simulink model "simModel2020"  (R2023b)
settings: Solver=ode4  StartTime=0  StopTime=360  FixedStep=0.01  RelTol=1e-3
values from neighbouring files (symbols this model uses):
  B747 =     [B747.mat]
undefined symbols (not defined in the file or in its folder): airport, APP, control, Curise, Earth, env, ft, m, navData, navParam, Newton, plotTrack, Raphson, s, TakeOff, WGS84
libraries: aerolibconvert2 x18, simulink x15, sharedtransform x4, aerolibfltsims x3, aerolibatmos2 x2, shared6dof x2, aerolibasang x2, dspsrcs4 x2, aerolibwind2 x2, aerolibanimutils x1, aerolibpropulsion2 x1, aerolibtransform2 x1
(part 5 of 6)

== system simModel2020/AutoPilot/InnerLoopAutopilot/Longitudinal Channel经度通道/AutoThrottle/AT Mode = 5,Idle/Rate Limiter Dynamic with External IC and Autoreset for Change in IC/Saturation Dynamic ==
  up : Inport
  u : Inport  Port=2
  lo : Inport  Port=3
  Data Type Duplicate : DataTypeDuplicate  DisableCoverage=on
  Data Type Propagation : S-Function  FunctionName=sfix_dtprop  Parameters=14,PropDataTypeMode,(getdatatypespecs(PropDataType,PropScaling,DblOver,0, 0, PropDataTypeMode, PropScalingMode)),IfRefDouble,IfRefSingle,IsSigned,NumBitsBase,NumBitsMult,NumBitsAdd,(sort(reshape(round(NumBitsAllowFinal), prod(size(NumBitsAllowFinal)),1))),PropScalingMode,ValuesUsedBestPrec,SlopeBase,SlopeMult,SlopeAdd,BiasBase,BiasMult,BiasAdd,DblOver  SFunctionDeploymentMode=off  EnableBusSupport=off  mask(Data Type Propagation){PropDataTypeMode=Inherit via propagation rule, PropDataType=fixdt(1, 16), IfRefDouble=double, IfRefSingle=single, IsSigned=IsSigned1, NumBitsBase=NumBits1, NumBitsMult=1, NumBitsAdd=0, NumBitsAllowFinal=1:128, PropScalingMode=Inherit via propagation rule, PropScaling=2^-10, ValuesUsedBestPrec=[5 -7], SlopeBase=Slope1, SlopeMult=1, SlopeAdd=0, BiasBase=Bias1, BiasMult=1, BiasAdd=0}
      mask prompts: PropDataTypeMode "Simulink:masks:x1PropagatedDataType_MP"; PropDataType "Simulink:masks:x11PropagatedDataTypeegFixdt116Fixdtsingle_MP"; IfRefDouble "Simulink:masks:x11IfAnyReferenceInputIsDoubleOutputIs_MP"; IfRefSingle "Simulink:masks:x12IfAnyReferenceInputIsSingleOutputIs_MP"; IsSigned "Simulink:masks:x13IsSigned_MP"; NumBitsBase "Simulink:masks:x141NumberofBitsBase_MP"; NumBitsMult "Simulink:masks:x142NumberofBitsMultiplicativeAdjustment_MP"; NumBitsAdd "Simulink:masks:x143NumberofBitsAdditiveAdjustment_MP"; NumBitsAllowFinal "Simulink:masks:x144NumberofBitsAllowableFinalValues_MP"; PropScalingMode "Simulink:masks:x2PropagatedScaling_MP"; PropScaling "Simulink:masks:x21PropagatedScalingSlopeEg29OrSlopeBiasEg1253_MP"; ValuesUsedBestPrec "Simulink:masks:x21ValuesUsedToDetermineBestPrecisionScaling_MP"; SlopeBase "Simulink:masks:x211SlopeBase_MP"; SlopeMult "Simulink:masks:x212SlopeMultiplicativeAdjustment_MP"; SlopeAdd "Simulink:masks:x213SlopeAdditiveAdjustment_MP"; BiasBase "Simulink:masks:x221BiasBase_MP"; BiasMult "Simulink:masks:x222BiasMultiplicativeAdjustment_MP"; BiasAdd "Simulink:masks:x223BiasAdditiveAdjustment_MP"
      mask help: Simulink:masks:DataTypePropagation_MD
      mask init:
      | DblOver = 0;
      mask TypeOptions PropDataTypeMode: Simulink:masks:SpecifyViaDialog | Simulink:masks:InheritViaPropagationRule
      mask Callback PropDataTypeMode: fixptdialog(gcbh)
      mask Callback PropDataType: fixptdialog(gcbh)
      mask TypeOptions IfRefDouble: Simulink:masks:double | Simulink:masks:single
      mask TypeOptions IfRefSingle: Simulink:masks:double | Simulink:masks:single
      mask TypeOptions IsSigned: Simulink:masks:IsSigned1 | Simulink:masks:IsSigned2 | Simulink:masks:IsSigned1OrIsSigned2 | Simulink:masks:TRUE | Simulink:masks:FALSE
      mask TypeOptions NumBitsBase: NumBits1 | NumBits2 | max([NumBits1 NumBits2]) | min([NumBits1 NumBits2]) | NumBits1+NumBits2
      mask TypeOptions PropScalingMode: Simulink:masks:SpecifyViaDialog | Simulink:masks:InheritViaPropagationRule | Simulink:masks:ObtainViaBestPrecision
      mask Callback PropScalingMode: fixptdialog(gcbh)
      mask TypeOptions SlopeBase: Slope1 | Slope2 | max([Slope1 Slope2]) | min([Slope1 Slope2]) | Slope1*Slope2 | Slope1/Slope2 | PosRange1 | PosRange2 | max([PosRange1 PosRange2]) | min([PosRange1 PosRange2]) | PosRange1*PosRange2 | PosRange1/PosRange2
      mask TypeOptions BiasBase: Bias1 | Bias2 | max([Bias1 Bias2]) | min([Bias1 Bias2]) | Bias1*Bias2 | Bias1/Bias2 | Bias1+Bias2 | Bias1-Bias2
      mask Display:
      | port_label('Input',1,'Ref1');
      | port_label('Input',2,'Ref2');
      | port_label('Input',3,'Prop');
  LowerRelop1 : RelationalOperator  DisableCoverage=on  Operator=>  OutDataTypeStr=boolean  InputSameDT=off
  Switch : Switch  Criteria=u2 ~= 0  OutDataTypeStr=Inherit: Inherit via back propagation  ZeroCross=off  SaturateOnIntegerOverflow=off  InputSameDT=off
  Switch2 : Switch  Criteria=u2 ~= 0  OutMin=OutMin  OutMax=OutMax  OutDataTypeStr=Inherit: Inherit via back propagation  ZeroCross=off  SaturateOnIntegerOverflow=off  InputSameDT=off
  UpperRelop : RelationalOperator  DisableCoverage=on  Operator=<  OutDataTypeStr=boolean  InputSameDT=off
  y : Outport  OutMin=OutMin  OutMax=OutMax
  wires:
  up/1 -> Switch2/1, LowerRelop1/2
  u/1 -> Data Type Propagation/2, Data Type Propagation/1, LowerRelop1/1, Switch/3, UpperRelop/1
  lo/1 -> Switch/1, UpperRelop/2
  Switch/1 -> Data Type Duplicate/2, Switch2/3, Data Type Propagation/3
  Switch2/1 -> Data Type Duplicate/1, y/1
  LowerRelop1/1 -> Switch2/2
  UpperRelop/1 -> Switch/2

== system simModel2020/AutoPilot/InnerLoopAutopilot/Longitudinal Channel经度通道/AutoThrottle/AT Mode = 5,Idle/Rate Limiter Dynamic with External IC and Autoreset for Change in IC/Subsystem ==
  WP Fly : Inport
  Compare To Constant : Subsystem  mask(Compare To Constant){relop=>=, const=0.5, OutDataTypeStr=boolean, ZeroCross=on}
      mask prompts: relop "Simulink:masks:Operator_MP"; const "Simulink:masks:ConstantValue_MP"; OutDataTypeStr "Simulink:masks:OutputDataType_MP"; ZeroCross "Simulink:masks:EnableZerocrossingDetection_MP"
      mask help: Simulink:masks:CompareToConstant_MD
      mask init: same as simModel2020/AutoPilot/InnerLoopAutopilot/Longitudinal Channel经度通道/AutoThrottle/AT Mode = 0,Recycle/Rate Limiter Dynamic with External IC and Autoreset for Change in IC/Subsystem/Compare To Constant
      mask TypeOptions relop: == | ~= | < | <= | >= | >
      mask TypeOptions OutDataTypeStr: Simulink:masks:uint8 | Simulink:masks:boolean
      mask Callback ZeroCross: sl('zeroCrossEnable', gcbh);
      mask Display: disp(str)
  Compare To Constant1 : Subsystem  mask(Compare To Constant){relop=<, const=0.5, OutDataTypeStr=boolean, ZeroCross=on}
      mask prompts: relop "Simulink:masks:Operator_MP"; const "Simulink:masks:ConstantValue_MP"; OutDataTypeStr "Simulink:masks:OutputDataType_MP"; ZeroCross "Simulink:masks:EnableZerocrossingDetection_MP"
      mask help: Simulink:masks:CompareToConstant_MD
      mask init: same as simModel2020/AutoPilot/InnerLoopAutopilot/Longitudinal Channel经度通道/AutoThrottle/AT Mode = 0,Recycle/Rate Limiter Dynamic with External IC and Autoreset for Change in IC/Subsystem/Compare To Constant
      mask TypeOptions relop: == | ~= | < | <= | >= | >
      mask TypeOptions OutDataTypeStr: Simulink:masks:uint8 | Simulink:masks:boolean
      mask Callback ZeroCross: sl('zeroCrossEnable', gcbh);
      mask Display: disp(str)
  Logical Operator : Logic  AllPortsSameDT=off  OutDataTypeStr=boolean
  Unit Delay : UnitDelay  SampleTime=-1  HasFrameUpgradeWarning=on
  Just Enab : Outport
  wires:
  WP Fly/1 -> Unit Delay/1, Compare To Constant/1(u)
  Compare To Constant/1(y) -> Logical Operator/1
  Compare To Constant1/1(y) -> Logical Operator/2
  Unit Delay/1 -> Compare To Constant1/1(u)
  Logical Operator/1 -> Just Enab/1

== system simModel2020/AutoPilot/InnerLoopAutopilot/Longitudinal Channel经度通道/AutoThrottle/AT Mode = 5,Idle/Rate Limiter Dynamic with External IC and Autoreset for Change in IC/Unit Delay Resettable External IC ==
  note: Reset
  note: Initial Value
  u : Inport
  R : Inport  Port=2
  IC : Inport  Port=3
  FixPt Constant : Constant  DisableCoverage=on  Value=0  OutDataTypeStr=fixdt(0,8,0)
  FixPt Data Type Duplicate1 : DataTypeDuplicate  DisableCoverage=on  NumInputPorts=4
  FixPt Logical Operator : Logic  DisableCoverage=on  Operator=OR  AllPortsSameDT=off  OutDataTypeStr=fixdt(0, 8)
  FixPt Unit Delay1 : UnitDelay  DisableCoverage=on  InitialCondition=0.0  SampleTime=tsamp
  FixPt Unit Delay2 : UnitDelay  DisableCoverage=on  InitialCondition=1  SampleTime=tsamp  HasFrameUpgradeWarning=on
  Init : Switch  Criteria=u2 ~= 0  OutDataTypeStr=Inherit: Inherit via back propagation  ZeroCross=off  SaturateOnIntegerOverflow=off  InputSameDT=off
  Reset : Switch  Criteria=u2 ~= 0  OutDataTypeStr=Inherit: Inherit via back propagation  ZeroCross=off  SaturateOnIntegerOverflow=off  InputSameDT=off
  State Control : Subsystem  Description=Replaced Block  mask(Replaced Block){}
      mask help: This block has been replaced with an empty subsystem because it used functionality that is unavailable in Simulink R2014a.
      mask Display: fprintf('Replaced: %s\n','StateControl')
  y : Outport
  wires:
  FixPt Logical Operator/1 -> Init/2
  FixPt Unit Delay1/1 -> Init/3  "Xold"
  Init/1 -> y/1, FixPt Data Type Duplicate1/1
  FixPt Unit Delay2/1 -> FixPt Logical Operator/2
  FixPt Constant/1 -> FixPt Unit Delay2/1
  R/1 -> FixPt Logical Operator/1, Reset/2
  Reset/1 -> FixPt Unit Delay1/1, FixPt Data Type Duplicate1/2  "Xnew"
  u/1 -> Reset/3, FixPt Data Type Duplicate1/4
  IC/1 -> FixPt Data Type Duplicate1/3, Init/1, Reset/1

== system simModel2020/AutoPilot/InnerLoopAutopilot/Longitudinal Channel经度通道/PitchStyle/Altitude Hold/Filter1/Subsystem ==
  In : Inport
  Enable : EnablePort  StatesWhenEnabling=reset
  " " : Outport  InitialOutput=0
  wires:
  In/1 -> " "/1

== system simModel2020/AutoPilot/InnerLoopAutopilot/Longitudinal Channel经度通道/PitchStyle/IAS_Control_dE/Filter2/Subsystem ==
  In : Inport
  Enable : EnablePort  StatesWhenEnabling=reset
  " " : Outport  InitialOutput=0
  wires:
  In/1 -> " "/1

== system simModel2020/AutoPilot/InnerLoopAutopilot/Longitudinal Channel经度通道/PitchStyle/Pitch Control/Filter2/Subsystem ==
  In : Inport
  Enable : EnablePort  StatesWhenEnabling=reset
  " " : Outport  InitialOutput=0
  wires:
  In/1 -> " "/1

== system simModel2020/AutoPilot/InnerLoopAutopilot/Longitudinal Channel经度通道/PitchStyle/Rate Limiter Dynamic/Rate Limiter Dynamic with External IC and Autoreset for Change in IC1/Saturation Dynamic ==
  up : Inport
  u : Inport  Port=2
  lo : Inport  Port=3
  Data Type Duplicate : DataTypeDuplicate  DisableCoverage=on
  Data Type Propagation : S-Function  FunctionName=sfix_dtprop  Parameters=14,PropDataTypeMode,(getdatatypespecs(PropDataType,PropScaling,DblOver,0, 0, PropDataTypeMode, PropScalingMode)),IfRefDouble,IfRefSingle,IsSigned,NumBitsBase,NumBitsMult,NumBitsAdd,(sort(reshape(round(NumBitsAllowFinal), prod(size(NumBitsAllowFinal)),1))),PropScalingMode,ValuesUsedBestPrec,SlopeBase,SlopeMult,SlopeAdd,BiasBase,BiasMult,BiasAdd,DblOver  SFunctionDeploymentMode=off  EnableBusSupport=off  mask(Data Type Propagation){PropDataTypeMode=Inherit via propagation rule, PropDataType=fixdt(1, 16), IfRefDouble=double, IfRefSingle=single, IsSigned=IsSigned1, NumBitsBase=NumBits1, NumBitsMult=1, NumBitsAdd=0, NumBitsAllowFinal=1:128, PropScalingMode=Inherit via propagation rule, PropScaling=2^-10, ValuesUsedBestPrec=[5 -7], SlopeBase=Slope1, SlopeMult=1, SlopeAdd=0, BiasBase=Bias1, BiasMult=1, BiasAdd=0}
      mask prompts: PropDataTypeMode "Simulink:masks:x1PropagatedDataType_MP"; PropDataType "Simulink:masks:x11PropagatedDataTypeegFixdt116Fixdtsingle_MP"; IfRefDouble "Simulink:masks:x11IfAnyReferenceInputIsDoubleOutputIs_MP"; IfRefSingle "Simulink:masks:x12IfAnyReferenceInputIsSingleOutputIs_MP"; IsSigned "Simulink:masks:x13IsSigned_MP"; NumBitsBase "Simulink:masks:x141NumberofBitsBase_MP"; NumBitsMult "Simulink:masks:x142NumberofBitsMultiplicativeAdjustment_MP"; NumBitsAdd "Simulink:masks:x143NumberofBitsAdditiveAdjustment_MP"; NumBitsAllowFinal "Simulink:masks:x144NumberofBitsAllowableFinalValues_MP"; PropScalingMode "Simulink:masks:x2PropagatedScaling_MP"; PropScaling "Simulink:masks:x21PropagatedScalingSlopeEg29OrSlopeBiasEg1253_MP"; ValuesUsedBestPrec "Simulink:masks:x21ValuesUsedToDetermineBestPrecisionScaling_MP"; SlopeBase "Simulink:masks:x211SlopeBase_MP"; SlopeMult "Simulink:masks:x212SlopeMultiplicativeAdjustment_MP"; SlopeAdd "Simulink:masks:x213SlopeAdditiveAdjustment_MP"; BiasBase "Simulink:masks:x221BiasBase_MP"; BiasMult "Simulink:masks:x222BiasMultiplicativeAdjustment_MP"; BiasAdd "Simulink:masks:x223BiasAdditiveAdjustment_MP"
      mask help: Simulink:masks:DataTypePropagation_MD
      mask init:
      | DblOver = 0;
      mask TypeOptions PropDataTypeMode: Simulink:masks:SpecifyViaDialog | Simulink:masks:InheritViaPropagationRule
      mask Callback PropDataTypeMode: fixptdialog(gcbh)
      mask Callback PropDataType: fixptdialog(gcbh)
      mask TypeOptions IfRefDouble: Simulink:masks:double | Simulink:masks:single
      mask TypeOptions IfRefSingle: Simulink:masks:double | Simulink:masks:single
      mask TypeOptions IsSigned: Simulink:masks:IsSigned1 | Simulink:masks:IsSigned2 | Simulink:masks:IsSigned1OrIsSigned2 | Simulink:masks:TRUE | Simulink:masks:FALSE
      mask TypeOptions NumBitsBase: NumBits1 | NumBits2 | max([NumBits1 NumBits2]) | min([NumBits1 NumBits2]) | NumBits1+NumBits2
      mask TypeOptions PropScalingMode: Simulink:masks:SpecifyViaDialog | Simulink:masks:InheritViaPropagationRule | Simulink:masks:ObtainViaBestPrecision
      mask Callback PropScalingMode: fixptdialog(gcbh)
      mask TypeOptions SlopeBase: Slope1 | Slope2 | max([Slope1 Slope2]) | min([Slope1 Slope2]) | Slope1*Slope2 | Slope1/Slope2 | PosRange1 | PosRange2 | max([PosRange1 PosRange2]) | min([PosRange1 PosRange2]) | PosRange1*PosRange2 | PosRange1/PosRange2
      mask TypeOptions BiasBase: Bias1 | Bias2 | max([Bias1 Bias2]) | min([Bias1 Bias2]) | Bias1*Bias2 | Bias1/Bias2 | Bias1+Bias2 | Bias1-Bias2
      mask Display:
      | port_label('Input',1,'Ref1');
      | port_label('Input',2,'Ref2');
      | port_label('Input',3,'Prop');
  LowerRelop1 : RelationalOperator  DisableCoverage=on  Operator=>  OutDataTypeStr=boolean  InputSameDT=off
  Switch : Switch  Criteria=u2 ~= 0  OutDataTypeStr=Inherit: Inherit via back propagation  ZeroCross=off  SaturateOnIntegerOverflow=off  InputSameDT=off
  Switch2 : Switch  Criteria=u2 ~= 0  OutMin=OutMin  OutMax=OutMax  OutDataTypeStr=Inherit: Inherit via back propagation  ZeroCross=off  SaturateOnIntegerOverflow=off  InputSameDT=off
  UpperRelop : RelationalOperator  DisableCoverage=on  Operator=<  OutDataTypeStr=boolean  InputSameDT=off
  y : Outport  OutMin=OutMin  OutMax=OutMax
  wires:
  UpperRelop/1 -> Switch/2
  LowerRelop1/1 -> Switch2/2
  Switch2/1 -> y/1, Data Type Duplicate/1
  Switch/1 -> Data Type Propagation/3, Switch2/3, Data Type Duplicate/2
  lo/1 -> UpperRelop/2, Switch/1
  u/1 -> UpperRelop/1, Switch/3, LowerRelop1/1, Data Type Propagation/1, Data Type Propagation/2
  up/1 -> LowerRelop1/2, Switch2/1

== system simModel2020/AutoPilot/InnerLoopAutopilot/Longitudinal Channel经度通道/PitchStyle/Rate Limiter Dynamic/Rate Limiter Dynamic with External IC and Autoreset for Change in IC1/Subsystem ==
  WP Fly : Inport
  Compare To Constant : Subsystem  mask(Compare To Constant){relop=>=, const=0.5, OutDataTypeStr=boolean, ZeroCross=on}
      mask prompts: relop "Simulink:masks:Operator_MP"; const "Simulink:masks:ConstantValue_MP"; OutDataTypeStr "Simulink:masks:OutputDataType_MP"; ZeroCross "Simulink:masks:EnableZerocrossingDetection_MP"
      mask help: Simulink:masks:CompareToConstant_MD
      mask init: same as simModel2020/AutoPilot/InnerLoopAutopilot/Longitudinal Channel经度通道/AutoThrottle/AT Mode = 0,Recycle/Rate Limiter Dynamic with External IC and Autoreset for Change in IC/Subsystem/Compare To Constant
      mask TypeOptions relop: == | ~= | < | <= | >= | >
      mask TypeOptions OutDataTypeStr: Simulink:masks:uint8 | Simulink:masks:boolean
      mask Callback ZeroCross: sl('zeroCrossEnable', gcbh);
      mask Display: disp(str)
  Compare To Constant1 : Subsystem  mask(Compare To Constant){relop=<, const=0.5, OutDataTypeStr=boolean, ZeroCross=on}
      mask prompts: relop "Simulink:masks:Operator_MP"; const "Simulink:masks:ConstantValue_MP"; OutDataTypeStr "Simulink:masks:OutputDataType_MP"; ZeroCross "Simulink:masks:EnableZerocrossingDetection_MP"
      mask help: Simulink:masks:CompareToConstant_MD
      mask init: same as simModel2020/AutoPilot/InnerLoopAutopilot/Longitudinal Channel经度通道/AutoThrottle/AT Mode = 0,Recycle/Rate Limiter Dynamic with External IC and Autoreset for Change in IC/Subsystem/Compare To Constant
      mask TypeOptions relop: == | ~= | < | <= | >= | >
      mask TypeOptions OutDataTypeStr: Simulink:masks:uint8 | Simulink:masks:boolean
      mask Callback ZeroCross: sl('zeroCrossEnable', gcbh);
      mask Display: disp(str)
  Logical Operator : Logic  AllPortsSameDT=off  OutDataTypeStr=boolean
  Unit Delay : UnitDelay  SampleTime=-1  HasFrameUpgradeWarning=on
  Just Enab : Outport
  wires:
  Logical Operator/1 -> Just Enab/1
  Unit Delay/1 -> Compare To Constant1/1(u)
  Compare To Constant1/1(y) -> Logical Operator/2
  Compare To Constant/1(y) -> Logical Operator/1
  WP Fly/1 -> Compare To Constant/1(u), Unit Delay/1

== system simModel2020/AutoPilot/InnerLoopAutopilot/Longitudinal Channel经度通道/PitchStyle/Rate Limiter Dynamic/Rate Limiter Dynamic with External IC and Autoreset for Change in IC1/Unit Delay Resettable External IC ==
  note: Initial Value
  note: Reset
  u : Inport
  R : Inport  Port=2
  IC : Inport  Port=3
  FixPt Constant : Constant  DisableCoverage=on  Value=0  OutDataTypeStr=fixdt(0,8,0)
  FixPt Data Type Duplicate1 : DataTypeDuplicate  DisableCoverage=on  NumInputPorts=4
  FixPt Logical Operator : Logic  DisableCoverage=on  Operator=OR  AllPortsSameDT=off  OutDataTypeStr=fixdt(0, 8)
  FixPt Unit Delay1 : UnitDelay  DisableCoverage=on  InitialCondition=0.0  SampleTime=tsamp
  FixPt Unit Delay2 : UnitDelay  DisableCoverage=on  InitialCondition=1  SampleTime=tsamp  HasFrameUpgradeWarning=on
  Init : Switch  Criteria=u2 ~= 0  OutDataTypeStr=Inherit: Inherit via back propagation  ZeroCross=off  SaturateOnIntegerOverflow=off  InputSameDT=off
  Reset : Switch  Criteria=u2 ~= 0  OutDataTypeStr=Inherit: Inherit via back propagation  ZeroCross=off  SaturateOnIntegerOverflow=off  InputSameDT=off
  State Control : Subsystem  Description=Replaced Block  mask(Replaced Block){}
      mask help: This block has been replaced with an empty subsystem because it used functionality that is unavailable in Simulink R2014a.
      mask Display: fprintf('Replaced: %s\n','StateControl')
  y : Outport
  wires:
  IC/1 -> Reset/1, Init/1, FixPt Data Type Duplicate1/3
  u/1 -> FixPt Data Type Duplicate1/4, Reset/3
  Reset/1 -> FixPt Data Type Duplicate1/2, FixPt Unit Delay1/1  "Xnew"
  R/1 -> Reset/2, FixPt Logical Operator/1
  FixPt Constant/1 -> FixPt Unit Delay2/1
  FixPt Unit Delay2/1 -> FixPt Logical Operator/2
  Init/1 -> FixPt Data Type Duplicate1/1, y/1
  FixPt Unit Delay1/1 -> Init/3  "Xold"
  FixPt Logical Operator/1 -> Init/2

== system simModel2020/AutoPilot/InnerLoopAutopilot/Longitudinal Channel经度通道/PitchStyle/Rate Limiter Dynamic/Sample(1//z)/Detect Change ==
  note: Edge
  note: U(k)
  U : Inport
  Delay Input1 : UnitDelay  Description=Store in Global RAM  DisableCoverage=on  InitialCondition=vinit  SampleTime=-1  HasFrameUpgradeWarning=on
  FixPt Relational Operator : RelationalOperator  Operator=~=  OutDataTypeStr=boolean  ZeroCross=off  InputSameDT=off
  Y : Outport  InitialOutput=0
  wires:
  FixPt Relational Operator/1 -> Y/1
  Delay Input1/1 -> FixPt Relational Operator/2  "U(k-1)"
  U/1 -> FixPt Relational Operator/1, Delay Input1/1

== system simModel2020/AutoPilot/InnerLoopAutopilot/Longitudinal Channel经度通道/PitchStyle/Rate Limiter Dynamic/Sample(1//z)/Sample and Hold ==
  In : Inport
  Trigger : TriggerPort  TriggerType=either  VariantControl=Variant  ZeroCross=off
  " " : Outport  InitialOutput=initCond
  wires:
  In/1 -> " "/1

== system simModel2020/AutoPilot/InnerLoopAutopilot/Longitudinal Channel经度通道/PitchStyle/Rate Limiter Dynamic1/Rate Limiter Dynamic with External IC and Autoreset for Change in IC/Saturation Dynamic ==
  up : Inport
  u : Inport  Port=2
  lo : Inport  Port=3
  Data Type Duplicate : DataTypeDuplicate  DisableCoverage=on
  Data Type Propagation : S-Function  FunctionName=sfix_dtprop  Parameters=14,PropDataTypeMode,(getdatatypespecs(PropDataType,PropScaling,DblOver,0, 0, PropDataTypeMode, PropScalingMode)),IfRefDouble,IfRefSingle,IsSigned,NumBitsBase,NumBitsMult,NumBitsAdd,(sort(reshape(round(NumBitsAllowFinal), prod(size(NumBitsAllowFinal)),1))),PropScalingMode,ValuesUsedBestPrec,SlopeBase,SlopeMult,SlopeAdd,BiasBase,BiasMult,BiasAdd,DblOver  SFunctionDeploymentMode=off  EnableBusSupport=off  mask(Data Type Propagation){PropDataTypeMode=Inherit via propagation rule, PropDataType=fixdt(1, 16), IfRefDouble=double, IfRefSingle=single, IsSigned=IsSigned1, NumBitsBase=NumBits1, NumBitsMult=1, NumBitsAdd=0, NumBitsAllowFinal=1:128, PropScalingMode=Inherit via propagation rule, PropScaling=2^-10, ValuesUsedBestPrec=[5 -7], SlopeBase=Slope1, SlopeMult=1, SlopeAdd=0, BiasBase=Bias1, BiasMult=1, BiasAdd=0}
      mask prompts: PropDataTypeMode "Simulink:masks:x1PropagatedDataType_MP"; PropDataType "Simulink:masks:x11PropagatedDataTypeegFixdt116Fixdtsingle_MP"; IfRefDouble "Simulink:masks:x11IfAnyReferenceInputIsDoubleOutputIs_MP"; IfRefSingle "Simulink:masks:x12IfAnyReferenceInputIsSingleOutputIs_MP"; IsSigned "Simulink:masks:x13IsSigned_MP"; NumBitsBase "Simulink:masks:x141NumberofBitsBase_MP"; NumBitsMult "Simulink:masks:x142NumberofBitsMultiplicativeAdjustment_MP"; NumBitsAdd "Simulink:masks:x143NumberofBitsAdditiveAdjustment_MP"; NumBitsAllowFinal "Simulink:masks:x144NumberofBitsAllowableFinalValues_MP"; PropScalingMode "Simulink:masks:x2PropagatedScaling_MP"; PropScaling "Simulink:masks:x21PropagatedScalingSlopeEg29OrSlopeBiasEg1253_MP"; ValuesUsedBestPrec "Simulink:masks:x21ValuesUsedToDetermineBestPrecisionScaling_MP"; SlopeBase "Simulink:masks:x211SlopeBase_MP"; SlopeMult "Simulink:masks:x212SlopeMultiplicativeAdjustment_MP"; SlopeAdd "Simulink:masks:x213SlopeAdditiveAdjustment_MP"; BiasBase "Simulink:masks:x221BiasBase_MP"; BiasMult "Simulink:masks:x222BiasMultiplicativeAdjustment_MP"; BiasAdd "Simulink:masks:x223BiasAdditiveAdjustment_MP"
      mask help: Simulink:masks:DataTypePropagation_MD
      mask init:
      | DblOver = 0;
      mask TypeOptions PropDataTypeMode: Simulink:masks:SpecifyViaDialog | Simulink:masks:InheritViaPropagationRule
      mask Callback PropDataTypeMode: fixptdialog(gcbh)
      mask Callback PropDataType: fixptdialog(gcbh)
      mask TypeOptions IfRefDouble: Simulink:masks:double | Simulink:masks:single
      mask TypeOptions IfRefSingle: Simulink:masks:double | Simulink:masks:single
      mask TypeOptions IsSigned: Simulink:masks:IsSigned1 | Simulink:masks:IsSigned2 | Simulink:masks:IsSigned1OrIsSigned2 | Simulink:masks:TRUE | Simulink:masks:FALSE
      mask TypeOptions NumBitsBase: NumBits1 | NumBits2 | max([NumBits1 NumBits2]) | min([NumBits1 NumBits2]) | NumBits1+NumBits2
      mask TypeOptions PropScalingMode: Simulink:masks:SpecifyViaDialog | Simulink:masks:InheritViaPropagationRule | Simulink:masks:ObtainViaBestPrecision
      mask Callback PropScalingMode: fixptdialog(gcbh)
      mask TypeOptions SlopeBase: Slope1 | Slope2 | max([Slope1 Slope2]) | min([Slope1 Slope2]) | Slope1*Slope2 | Slope1/Slope2 | PosRange1 | PosRange2 | max([PosRange1 PosRange2]) | min([PosRange1 PosRange2]) | PosRange1*PosRange2 | PosRange1/PosRange2
      mask TypeOptions BiasBase: Bias1 | Bias2 | max([Bias1 Bias2]) | min([Bias1 Bias2]) | Bias1*Bias2 | Bias1/Bias2 | Bias1+Bias2 | Bias1-Bias2
      mask Display:
      | port_label('Input',1,'Ref1');
      | port_label('Input',2,'Ref2');
      | port_label('Input',3,'Prop');
  LowerRelop1 : RelationalOperator  DisableCoverage=on  Operator=>  OutDataTypeStr=boolean  InputSameDT=off
  Switch : Switch  Criteria=u2 ~= 0  OutDataTypeStr=Inherit: Inherit via back propagation  ZeroCross=off  SaturateOnIntegerOverflow=off  InputSameDT=off
  Switch2 : Switch  Criteria=u2 ~= 0  OutMin=OutMin  OutMax=OutMax  OutDataTypeStr=Inherit: Inherit via back propagation  ZeroCross=off  SaturateOnIntegerOverflow=off  InputSameDT=off
  UpperRelop : RelationalOperator  DisableCoverage=on  Operator=<  OutDataTypeStr=boolean  InputSameDT=off
  y : Outport  OutMin=OutMin  OutMax=OutMax
  wires:
  up/1 -> Switch2/1, LowerRelop1/2
  u/1 -> Data Type Propagation/2, Data Type Propagation/1, LowerRelop1/1, Switch/3, UpperRelop/1
  lo/1 -> Switch/1, UpperRelop/2
  Switch/1 -> Data Type Duplicate/2, Switch2/3, Data Type Propagation/3
  Switch2/1 -> Data Type Duplicate/1, y/1
  LowerRelop1/1 -> Switch2/2
  UpperRelop/1 -> Switch/2

== system simModel2020/AutoPilot/InnerLoopAutopilot/Longitudinal Channel经度通道/PitchStyle/Rate Limiter Dynamic1/Rate Limiter Dynamic with External IC and Autoreset for Change in IC/Subsystem ==
  WP Fly : Inport
  Compare To Constant : Subsystem  mask(Compare To Constant){relop=>=, const=0.5, OutDataTypeStr=boolean, ZeroCross=on}
      mask prompts: relop "Simulink:masks:Operator_MP"; const "Simulink:masks:ConstantValue_MP"; OutDataTypeStr "Simulink:masks:OutputDataType_MP"; ZeroCross "Simulink:masks:EnableZerocrossingDetection_MP"
      mask help: Simulink:masks:CompareToConstant_MD
      mask init: same as simModel2020/AutoPilot/InnerLoopAutopilot/Longitudinal Channel经度通道/AutoThrottle/AT Mode = 0,Recycle/Rate Limiter Dynamic with External IC and Autoreset for Change in IC/Subsystem/Compare To Constant
      mask TypeOptions relop: == | ~= | < | <= | >= | >
      mask TypeOptions OutDataTypeStr: Simulink:masks:uint8 | Simulink:masks:boolean
      mask Callback ZeroCross: sl('zeroCrossEnable', gcbh);
      mask Display: disp(str)
  Compare To Constant1 : Subsystem  mask(Compare To Constant){relop=<, const=0.5, OutDataTypeStr=boolean, ZeroCross=on}
      mask prompts: relop "Simulink:masks:Operator_MP"; const "Simulink:masks:ConstantValue_MP"; OutDataTypeStr "Simulink:masks:OutputDataType_MP"; ZeroCross "Simulink:masks:EnableZerocrossingDetection_MP"
      mask help: Simulink:masks:CompareToConstant_MD
      mask init: same as simModel2020/AutoPilot/InnerLoopAutopilot/Longitudinal Channel经度通道/AutoThrottle/AT Mode = 0,Recycle/Rate Limiter Dynamic with External IC and Autoreset for Change in IC/Subsystem/Compare To Constant
      mask TypeOptions relop: == | ~= | < | <= | >= | >
      mask TypeOptions OutDataTypeStr: Simulink:masks:uint8 | Simulink:masks:boolean
      mask Callback ZeroCross: sl('zeroCrossEnable', gcbh);
      mask Display: disp(str)
  Logical Operator : Logic  AllPortsSameDT=off  OutDataTypeStr=boolean
  Unit Delay : UnitDelay  SampleTime=-1  HasFrameUpgradeWarning=on
  Just Enab : Outport
  wires:
  WP Fly/1 -> Unit Delay/1, Compare To Constant/1(u)
  Compare To Constant/1(y) -> Logical Operator/1
  Compare To Constant1/1(y) -> Logical Operator/2
  Unit Delay/1 -> Compare To Constant1/1(u)
  Logical Operator/1 -> Just Enab/1

== system simModel2020/AutoPilot/InnerLoopAutopilot/Longitudinal Channel经度通道/PitchStyle/Rate Limiter Dynamic1/Rate Limiter Dynamic with External IC and Autoreset for Change in IC/Unit Delay Resettable External IC ==
  note: Reset
  note: Initial Value
  u : Inport
  R : Inport  Port=2
  IC : Inport  Port=3
  FixPt Constant : Constant  DisableCoverage=on  Value=0  OutDataTypeStr=fixdt(0,8,0)
  FixPt Data Type Duplicate1 : DataTypeDuplicate  DisableCoverage=on  NumInputPorts=4
  FixPt Logical Operator : Logic  DisableCoverage=on  Operator=OR  AllPortsSameDT=off  OutDataTypeStr=fixdt(0, 8)
  FixPt Unit Delay1 : UnitDelay  DisableCoverage=on  InitialCondition=0.0  SampleTime=tsamp
  FixPt Unit Delay2 : UnitDelay  DisableCoverage=on  InitialCondition=1  SampleTime=tsamp  HasFrameUpgradeWarning=on
  Init : Switch  Criteria=u2 ~= 0  OutDataTypeStr=Inherit: Inherit via back propagation  ZeroCross=off  SaturateOnIntegerOverflow=off  InputSameDT=off
  Reset : Switch  Criteria=u2 ~= 0  OutDataTypeStr=Inherit: Inherit via back propagation  ZeroCross=off  SaturateOnIntegerOverflow=off  InputSameDT=off
  State Control : Subsystem  Description=Replaced Block  mask(Replaced Block){}
      mask help: This block has been replaced with an empty subsystem because it used functionality that is unavailable in Simulink R2014a.
      mask Display: fprintf('Replaced: %s\n','StateControl')
  y : Outport
  wires:
  FixPt Logical Operator/1 -> Init/2
  FixPt Unit Delay1/1 -> Init/3  "Xold"
  Init/1 -> y/1, FixPt Data Type Duplicate1/1
  FixPt Unit Delay2/1 -> FixPt Logical Operator/2
  FixPt Constant/1 -> FixPt Unit Delay2/1
  R/1 -> FixPt Logical Operator/1, Reset/2
  Reset/1 -> FixPt Unit Delay1/1, FixPt Data Type Duplicate1/2  "Xnew"
  u/1 -> Reset/3, FixPt Data Type Duplicate1/4
  IC/1 -> FixPt Data Type Duplicate1/3, Init/1, Reset/1

== system simModel2020/AutoPilot/InnerLoopAutopilot/Longitudinal Channel经度通道/PitchStyle/Rate Limiter Dynamic1/Sample(1//z)/Detect Change ==
  note: Edge
  note: U(k)
  U : Inport
  Delay Input1 : UnitDelay  Description=Store in Global RAM  DisableCoverage=on  InitialCondition=vinit  SampleTime=-1  HasFrameUpgradeWarning=on
  FixPt Relational Operator : RelationalOperator  Operator=~=  OutDataTypeStr=boolean  ZeroCross=off  InputSameDT=off
  Y : Outport  InitialOutput=0
  wires:
  FixPt Relational Operator/1 -> Y/1
  Delay Input1/1 -> FixPt Relational Operator/2  "U(k-1)"
  U/1 -> FixPt Relational Operator/1, Delay Input1/1

== system simModel2020/AutoPilot/InnerLoopAutopilot/Longitudinal Channel经度通道/PitchStyle/Rate Limiter Dynamic1/Sample(1//z)/Sample and Hold ==
  In : Inport
  Trigger : TriggerPort  TriggerType=either  VariantControl=Variant  ZeroCross=off
  " " : Outport  InitialOutput=initCond
  wires:
  In/1 -> " "/1

== system simModel2020/AutoPilot/InnerLoopAutopilot/Longitudinal Channel经度通道/PitchStyle/Vtertical Speed Control/Filter1/Subsystem ==
  In : Inport
  Enable : EnablePort  StatesWhenEnabling=reset
  " " : Outport  InitialOutput=0
  wires:
  In/1 -> " "/1

== system simModel2020/PlantModel/B747 Dynamics动力学参数计算/Forces and Moments动力学计算/Compute Body Frame Forces and Moments气动力和力矩/Rotate FM to body frame/Rotate Forces/RB2W ==
  aoa beta : Inport
  11 : Fcn  Expr=u[3]*u[4]
  12 : Fcn  Expr=u[2]
  13 : Fcn  Expr=u[1]*u[4]
  21 : Fcn  Expr=-u[3]*u[2]
  22 : Fcn  Expr=u[4]
  23 : Fcn  Expr=-u[1]*u[2]
  31 : Fcn  Expr=-u[1]
  32 : Fcn  Expr=0
  33 : Fcn  Expr=u[3]
  Mux : Mux  Inputs=2
  Mux3 : Mux  Inputs=9
  Reshape 9x1->3x3 : Reshape  OutputDimensionality=Customize  OutputDimensions=[3,3]
  sincos : Trigonometry  Operator=sincos
  Rw2b : Outport
  wires:
  Mux/1 -> 11/1, 21/1, 31/1, 12/1, 22/1, 32/1, 13/1, 23/1, 33/1
  aoa beta/1 -> sincos/1
  sincos/2 -> Mux/2
  sincos/1 -> Mux/1
  33/1 -> Mux3/9
  23/1 -> Mux3/8
  13/1 -> Mux3/7
  32/1 -> Mux3/6
  22/1 -> Mux3/5
  12/1 -> Mux3/4
  31/1 -> Mux3/3
  21/1 -> Mux3/2
  11/1 -> Mux3/1
  Reshape 9x1->3x3/1 -> Rw2b/1
  Mux3/1 -> Reshape 9x1->3x3/1

== system simModel2020/PlantModel/B747 Dynamics动力学参数计算/Forces and Moments动力学计算/Compute Body Frame Forces and Moments气动力和力矩/Rotate FM to body frame/Rotate Moments/RB2W ==
  aoa beta : Inport
  11 : Fcn  Expr=u[3]*u[4]
  12 : Fcn  Expr=u[2]
  13 : Fcn  Expr=u[1]*u[4]
  21 : Fcn  Expr=-u[3]*u[2]
  22 : Fcn  Expr=u[4]
  23 : Fcn  Expr=-u[1]*u[2]
  31 : Fcn  Expr=-u[1]
  32 : Fcn  Expr=0
  33 : Fcn  Expr=u[3]
  Mux : Mux  Inputs=2
  Mux3 : Mux  Inputs=9
  Reshape 9x1->3x3 : Reshape  OutputDimensionality=Customize  OutputDimensions=[3,3]
  sincos : Trigonometry  Operator=sincos
  Rw2b : Outport
  wires:
  Mux/1 -> 11/1, 21/1, 31/1, 12/1, 22/1, 32/1, 13/1, 23/1, 33/1
  aoa beta/1 -> sincos/1
  sincos/2 -> Mux/2
  sincos/1 -> Mux/1
  33/1 -> Mux3/9
  23/1 -> Mux3/8
  13/1 -> Mux3/7
  32/1 -> Mux3/6
  22/1 -> Mux3/5
  12/1 -> Mux3/4
  31/1 -> Mux3/3
  21/1 -> Mux3/2
  11/1 -> Mux3/1
  Reshape 9x1->3x3/1 -> Rw2b/1
  Mux3/1 -> Reshape 9x1->3x3/1

== system simModel2020/PlantModel/B747 Dynamics动力学参数计算/Forces and Moments动力学计算/Compute Body Frame Forces and Moments气动力和力矩/Wind frame F& M 气动力计算/Lateral Channel/CY ==
  beta : Inport
  dR : Inport  Port=2
  CYDr : Constant  Value=B747.aero.CYDr
      settings: AttributesFormatString=%<Value>
  CYb : Constant  Value=B747.aero.CYb
      settings: AttributesFormatString=%<Value>
  Product : Product  SaturateOnIntegerOverflow=on  OutDataTypeStr=Inherit: Same as first input
  Product1 : Product  SaturateOnIntegerOverflow=on  OutDataTypeStr=Inherit: Same as first input
  Sum2 : Sum  SaturateOnIntegerOverflow=on
  CY : Outport
  wires:
  Product1/1 -> Sum2/2
  dR/1 -> Product1/2
  CYDr/1 -> Product1/1
  Product/1 -> Sum2/1
  Sum2/1 -> CY/1
  beta/1 -> Product/2
  CYb/1 -> Product/1

== system simModel2020/PlantModel/B747 Dynamics动力学参数计算/Forces and Moments动力学计算/Compute Body Frame Forces and Moments气动力和力矩/Wind frame F& M 气动力计算/Lateral Channel/Cl ==
  beta : Inport
  dA : Inport  Port=2
  dR : Inport  Port=3
  p,q,r : Inport  Port=4
  Airspeed : Inport  Port=5
  Deviation On : Inport  Port=6
  ClDa : Constant  Value=B747.aero.ClDa
      settings: AttributesFormatString=%<Value>
  ClDr : Constant  Value=B747.aero.ClDr
      settings: AttributesFormatString=%<Value>
  Clb : Constant  Value=B747.aero.Clb
      settings: AttributesFormatString=%<Value>
  Gain : Gain  Gain=0.05
  Multiport Switch : MultiPortSwitch  DataPortOrder=Specify indices  Inputs=2  DataPortIndices={1,0}  SaturateOnIntegerOverflow=off  InputSameDT=off
  Product1 : Product  SaturateOnIntegerOverflow=on  OutDataTypeStr=Inherit: Same as first input
  Product4 : Product  SaturateOnIntegerOverflow=on  OutDataTypeStr=Inherit: Same as first input
  Product5 : Product  SaturateOnIntegerOverflow=on  OutDataTypeStr=Inherit: Same as first input
  Sum : Sum  Inputs=+++++  SaturateOnIntegerOverflow=on
  Sum1 : Sum  Inputs=|++
  roll factors : Subsystem
  Cl : Outport
  wires:
  roll factors/1(Clp) -> Sum/4
  Product5/1 -> Gain/1, Sum1/2, Multiport Switch/3  "CldA"
  Airspeed/1 -> roll factors/2(Airspeed)
  p,q,r/1 -> roll factors/1(p,q,r)
  roll factors/2(Clr) -> Sum/5
  Product1/1 -> Sum/3  "Cldr"
  Product4/1 -> Sum/1  "Clb"
  Sum/1 -> Cl/1
  dR/1 -> Product1/2
  ClDr/1 -> Product1/1
  dA/1 -> Product5/2
  ClDa/1 -> Product5/1
  beta/1 -> Product4/2
  Clb/1 -> Product4/1
  Sum1/1 -> Multiport Switch/2
  Gain/1 -> Sum1/1
  Deviation On/1 -> Multiport Switch/1
  Multiport Switch/1 -> Sum/2

== system simModel2020/PlantModel/B747 Dynamics动力学参数计算/Forces and Moments动力学计算/Compute Body Frame Forces and Moments气动力和力矩/Wind frame F& M 气动力计算/Lateral Channel/Cn ==
  beta : Inport
  dA : Inport  Port=2
  Dr : Inport  Port=3
  p,q,r : Inport  Port=4
  Airspeed : Inport  Port=5
  CnDa : Constant  Value=B747.aero.CnDa
      settings: AttributesFormatString=%<Value>
  CnDr : Constant  Value=B747.aero.CnDr
      settings: AttributesFormatString=%<Value>
  Cnb : Constant  Value=B747.aero.Cnb
      settings: AttributesFormatString=%<Value>
  Product1 : Product  SaturateOnIntegerOverflow=on  OutDataTypeStr=Inherit: Same as first input
  Product4 : Product  SaturateOnIntegerOverflow=on  OutDataTypeStr=Inherit: Same as first input
  Product5 : Product  SaturateOnIntegerOverflow=on  OutDataTypeStr=Inherit: Same as first input
  Sum : Sum  Inputs=+++++  SaturateOnIntegerOverflow=on
  yaw factors : Subsystem
  Cn : Outport
  wires:
  Airspeed/1 -> yaw factors/2(Airspeed)
  p,q,r/1 -> yaw factors/1(p,q,r)
  Cnb/1 -> Product4/1
  beta/1 -> Product4/2
  CnDa/1 -> Product5/1
  Product5/1 -> Sum/2
  dA/1 -> Product5/2
  CnDr/1 -> Product1/1
  Dr/1 -> Product1/2
  Sum/1 -> Cn/1
  Product1/1 -> Sum/3
  yaw factors/2(Cnr) -> Sum/5
  yaw factors/1(Cnp) -> Sum/4
  Product4/1 -> Sum/1

== system simModel2020/PlantModel/B747 Dynamics动力学参数计算/Forces and Moments动力学计算/Compute Body Frame Forces and Moments气动力和力矩/Wind frame F& M 气动力计算/Longitudinal Channel/CD ==
  alpha : Inport
  Deviation On : Inport  Port=2
  Apolar (A2)1 : Constant  Value=B747.aero.CLa
      settings: AttributesFormatString=%<Value>
  Apolar (A2)2 : Constant  Value=B747.aero.CL0
      settings: AttributesFormatString=%<Value>
  Apolar (A2)3 : Constant  Value=pi*0.9*B747.geometry.span^2/B747.geometry.S
      settings: AttributesFormatString=%<Value>
  CD0 : Constant  Value=B747.aero.CDp
      settings: AttributesFormatString=%<Value>
  CD1 : Constant  Value=B747.aero.CD0
      settings: AttributesFormatString=%<Value>
  Divide : Product  Inputs=*/
  Gain : Gain  Gain=-1  SaturateOnIntegerOverflow=on  OutDataTypeStr=Inherit: Same as input  ParamDataTypeStr=Inherit: Same as input
      settings: AttributesFormatString=%<Gain>
  Gain1 : Gain  Gain=B747.aero.CDa
  Multiport Switch : MultiPortSwitch  DataPortOrder=Specify indices  Inputs=2  DataPortIndices={1,0}  SaturateOnIntegerOverflow=off  InputSameDT=off
  Product : Product
  Product1 : Product
  Sum : Sum  Inputs=|++
  Sum1 : Sum  Inputs=++|  SaturateOnIntegerOverflow=on
  Sum2 : Sum  Inputs=|++
  CD : Outport
  wires:
  Multiport Switch/1 -> Gain/1
  alpha/1 -> Gain1/1, Product1/1
  Sum1/1 -> Multiport Switch/2
  CD0/1 -> Sum1/1
  Apolar (A2)1/1 -> Product1/2
  Product1/1 -> Sum/1
  Apolar (A2)2/1 -> Sum/2
  Sum/1 -> Product/2, Product/1
  Product/1 -> Divide/1
  Apolar (A2)3/1 -> Divide/2
  Divide/1 -> Sum1/2
  CD1/1 -> Sum2/1
  Gain1/1 -> Sum2/2
  Sum2/1 -> Multiport Switch/3
  Deviation On/1 -> Multiport Switch/1
  Gain/1 -> CD/1

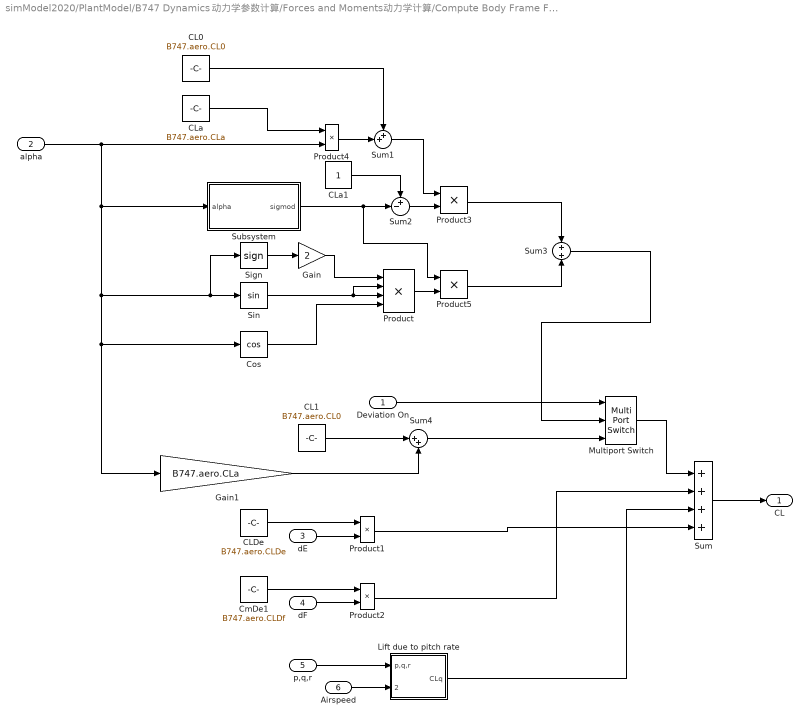
== system simModel2020/PlantModel/B747 Dynamics动力学参数计算/Forces and Moments动力学计算/Compute Body Frame Forces and Moments气动力和力矩/Wind frame F& M 气动力计算/Longitudinal Channel/CL ==
  Deviation On : Inport
  alpha : Inport  Port=2
  dE : Inport  Port=3
  dF : Inport  Port=4
  p,q,r : Inport  Port=5
  Airspeed : Inport  Port=6
  CL0 : Constant  Value=B747.aero.CL0
      settings: AttributesFormatString=%<Value>
  CL1 : Constant  Value=B747.aero.CL0
      settings: AttributesFormatString=%<Value>
  CLDe : Constant  Value=B747.aero.CLDe
      settings: AttributesFormatString=%<Value>
  CLa : Constant  Value=B747.aero.CLa
      settings: AttributesFormatString=%<Value>
  CLa1 : Constant
      settings: AttributesFormatString=%<Value>
  CmDe1 : Constant  Value=B747.aero.CLDf
      settings: AttributesFormatString=%<Value>
  Cos : Trigonometry  Operator=cos
  Gain : Gain  Gain=2
  Gain1 : Gain  Gain=B747.aero.CLa
  Lift due to pitch rate : Subsystem
  Multiport Switch : MultiPortSwitch  DataPortOrder=Specify indices  Inputs=2  DataPortIndices={1,0}  SaturateOnIntegerOverflow=off  InputSameDT=off
  Product : Product  Inputs=4
  Product1 : Product  SaturateOnIntegerOverflow=on  OutDataTypeStr=Inherit: Same as first input
  Product2 : Product  SaturateOnIntegerOverflow=on  OutDataTypeStr=Inherit: Same as first input
  Product3 : Product
  Product4 : Product  SaturateOnIntegerOverflow=on  OutDataTypeStr=Inherit: Same as first input
  Product5 : Product
  Sign : Signum
  Sin : Trigonometry
  Subsystem : Subsystem
  Sum : Sum  Inputs=++++  SaturateOnIntegerOverflow=on
  Sum1 : Sum  Inputs=++|
  Sum2 : Sum  Inputs=+-|
  Sum3 : Sum
  Sum4 : Sum  Inputs=|++
  CL : Outport
  wires:
  Airspeed/1 -> Lift due to pitch rate/2(Airspeed)
  p,q,r/1 -> Lift due to pitch rate/1(p,q,r)
  Lift due to pitch rate/1(CLq) -> Sum/3
  Product2/1 -> Sum/2
  Product1/1 -> Sum/4
  CmDe1/1 -> Product2/1
  dF/1 -> Product2/2
  Sum/1 -> CL/1
  dE/1 -> Product1/2
  CLDe/1 -> Product1/1
  alpha/1 -> Gain1/1, Cos/1, Sign/1, Sin/1, Subsystem/1(alpha), Product4/2
  CLa/1 -> Product4/1
  Product4/1 -> Sum1/2
  CL0/1 -> Sum1/1
  Sin/1 -> Product/3, Product/2
  Sign/1 -> Gain/1
  Gain/1 -> Product/1
  Cos/1 -> Product/4
  CLa1/1 -> Sum2/1
  Subsystem/1(sigmod) -> Product5/1, Sum2/2
  Sum2/1 -> Product3/2
  Sum1/1 -> Product3/1
  Product/1 -> Product5/2
  Product5/1 -> Sum3/2
  Product3/1 -> Sum3/1
  Sum3/1 -> Multiport Switch/2
  Multiport Switch/1 -> Sum/1
  CL1/1 -> Sum4/1
  Gain1/1 -> Sum4/2
  Sum4/1 -> Multiport Switch/3
  Deviation On/1 -> Multiport Switch/1

== system simModel2020/PlantModel/B747 Dynamics动力学参数计算/Forces and Moments动力学计算/Compute Body Frame Forces and Moments气动力和力矩/Wind frame F& M 气动力计算/Longitudinal Channel/Cm ==
  alpha : Inport
  dE : Inport  Port=2
  p,q,r : Inport  Port=3
  Airspeed : Inport  Port=4
  Deviation On : Inport  Port=5
  dF : Inport  Port=6
  Cm0 : Constant  Value=B747.aero.Cm0
      settings: AttributesFormatString=%<Value>
  CmDe : Constant  Value=B747.aero.CmDe
      settings: AttributesFormatString=%<Value>
  Cma : Constant  Value=B747.aero.Cma
      settings: AttributesFormatString=%<Value>
  Gain : Gain  Gain=0.05
  Gain1 : Gain  Gain=0.05
  Lift due to pitch rate : Subsystem
  Multiport Switch : MultiPortSwitch  DataPortOrder=Specify indices  Inputs=2  DataPortIndices={1,0}  SaturateOnIntegerOverflow=off  InputSameDT=off
  Multiport Switch1 : MultiPortSwitch  DataPortOrder=Specify indices  Inputs=2  DataPortIndices={1,0}  SaturateOnIntegerOverflow=off  InputSameDT=off
  Product1 : Product  Inputs=**  SaturateOnIntegerOverflow=on  OutDataTypeStr=Inherit: Same as first input
  Product4 : Product  SaturateOnIntegerOverflow=on  OutDataTypeStr=Inherit: Same as first input
  Sum : Sum  Inputs=++++  SaturateOnIntegerOverflow=on
  Sum1 : Sum  Inputs=|++
  Sum2 : Sum  Inputs=|++
  Terminator : Terminator
  Cm : Outport
  wires:
  Multiport Switch/1 -> Sum/4  "cmq"
  p,q,r/1 -> Lift due to pitch rate/1(p,q,r)
  Multiport Switch1/1 -> Sum/3  "cmde"
  Product4/1 -> Sum/2  "cma"
  Sum/1 -> Cm/1  "total"
  dE/1 -> Product1/2
  CmDe/1 -> Product1/1
  alpha/1 -> Product4/2
  Cma/1 -> Product4/1
  Cm0/1 -> Sum/1  "cm0"
  Airspeed/1 -> Lift due to pitch rate/2(Airspeed)
  Lift due to pitch rate/1(CMq) -> Gain/1, Sum1/2, Multiport Switch/3  "cmq"
  Gain/1 -> Sum1/1
  Sum1/1 -> Multiport Switch/2
  Deviation On/1 -> Multiport Switch1/1, Multiport Switch/1
  Product1/1 -> Gain1/1, Sum2/2, Multiport Switch1/3  "cmde"
  Gain1/1 -> Sum2/1
  Sum2/1 -> Multiport Switch1/2
  dF/1 -> Terminator/1

== system simModel2020/AutoPilot/InnerLoopAutopilot/Longitudinal Channel经度通道/AutoThrottle/AT Mode = 0,Recycle/Rate Limiter Dynamic with External IC and Autoreset for Change in IC/Subsystem/Compare To Constant ==
  u : Inport
  Compare : RelationalOperator  OutDataTypeStr=boolean
  Constant : Constant  DisableCoverage=on  Value=const  OutDataTypeStr=Inherit: Inherit via back propagation
  y : Outport
  wires:
  u/1 -> Compare/1
  Constant/1 -> Compare/2
  Compare/1 -> y/1

== system simModel2020/AutoPilot/InnerLoopAutopilot/Longitudinal Channel经度通道/AutoThrottle/AT Mode = 0,Recycle/Rate Limiter Dynamic with External IC and Autoreset for Change in IC/Subsystem/Compare To Constant1 ==
  u : Inport
  Compare : RelationalOperator  Operator=<  OutDataTypeStr=boolean
  Constant : Constant  DisableCoverage=on  Value=const  OutDataTypeStr=Inherit: Inherit via back propagation
  y : Outport
  wires:
  u/1 -> Compare/1
  Constant/1 -> Compare/2
  Compare/1 -> y/1

== system simModel2020/AutoPilot/InnerLoopAutopilot/Longitudinal Channel经度通道/AutoThrottle/AT Mode = 0,Recycle/Rate Limiter Dynamic with External IC and Autoreset for Change in IC/Unit Delay Resettable External IC/State Control ==

== system simModel2020/AutoPilot/InnerLoopAutopilot/Longitudinal Channel经度通道/AutoThrottle/AT Mode = 5,Idle/Rate Limiter Dynamic with External IC and Autoreset for Change in IC/Subsystem/Compare To Constant ==
  u : Inport
  Compare : RelationalOperator  OutDataTypeStr=boolean
  Constant : Constant  DisableCoverage=on  Value=const  OutDataTypeStr=Inherit: Inherit via back propagation
  y : Outport
  wires:
  u/1 -> Compare/1
  Constant/1 -> Compare/2
  Compare/1 -> y/1

== system simModel2020/AutoPilot/InnerLoopAutopilot/Longitudinal Channel经度通道/AutoThrottle/AT Mode = 5,Idle/Rate Limiter Dynamic with External IC and Autoreset for Change in IC/Subsystem/Compare To Constant1 ==
  u : Inport
  Compare : RelationalOperator  Operator=<  OutDataTypeStr=boolean
  Constant : Constant  DisableCoverage=on  Value=const  OutDataTypeStr=Inherit: Inherit via back propagation
  y : Outport
  wires:
  u/1 -> Compare/1
  Constant/1 -> Compare/2
  Compare/1 -> y/1

== system simModel2020/AutoPilot/InnerLoopAutopilot/Longitudinal Channel经度通道/AutoThrottle/AT Mode = 5,Idle/Rate Limiter Dynamic with External IC and Autoreset for Change in IC/Unit Delay Resettable External IC/State Control ==

== system simModel2020/AutoPilot/InnerLoopAutopilot/Longitudinal Channel经度通道/PitchStyle/Rate Limiter Dynamic/Rate Limiter Dynamic with External IC and Autoreset for Change in IC1/Subsystem/Compare To Constant ==
  u : Inport
  Compare : RelationalOperator  OutDataTypeStr=boolean
  Constant : Constant  DisableCoverage=on  Value=const  OutDataTypeStr=Inherit: Inherit via back propagation
  y : Outport
  wires:
  Compare/1 -> y/1
  Constant/1 -> Compare/2
  u/1 -> Compare/1

== system simModel2020/AutoPilot/InnerLoopAutopilot/Longitudinal Channel经度通道/PitchStyle/Rate Limiter Dynamic/Rate Limiter Dynamic with External IC and Autoreset for Change in IC1/Subsystem/Compare To Constant1 ==
  u : Inport
  Compare : RelationalOperator  Operator=<  OutDataTypeStr=boolean
  Constant : Constant  DisableCoverage=on  Value=const  OutDataTypeStr=Inherit: Inherit via back propagation
  y : Outport
  wires:
  Compare/1 -> y/1
  Constant/1 -> Compare/2
  u/1 -> Compare/1

== system simModel2020/AutoPilot/InnerLoopAutopilot/Longitudinal Channel经度通道/PitchStyle/Rate Limiter Dynamic/Rate Limiter Dynamic with External IC and Autoreset for Change in IC1/Unit Delay Resettable External IC/State Control ==

== system simModel2020/AutoPilot/InnerLoopAutopilot/Longitudinal Channel经度通道/PitchStyle/Rate Limiter Dynamic1/Rate Limiter Dynamic with External IC and Autoreset for Change in IC/Subsystem/Compare To Constant ==
  u : Inport
  Compare : RelationalOperator  OutDataTypeStr=boolean
  Constant : Constant  DisableCoverage=on  Value=const  OutDataTypeStr=Inherit: Inherit via back propagation
  y : Outport
  wires:
  u/1 -> Compare/1
  Constant/1 -> Compare/2
  Compare/1 -> y/1

== system simModel2020/AutoPilot/InnerLoopAutopilot/Longitudinal Channel经度通道/PitchStyle/Rate Limiter Dynamic1/Rate Limiter Dynamic with External IC and Autoreset for Change in IC/Subsystem/Compare To Constant1 ==
  u : Inport
  Compare : RelationalOperator  Operator=<  OutDataTypeStr=boolean
  Constant : Constant  DisableCoverage=on  Value=const  OutDataTypeStr=Inherit: Inherit via back propagation
  y : Outport
  wires:
  u/1 -> Compare/1
  Constant/1 -> Compare/2
  Compare/1 -> y/1

== system simModel2020/AutoPilot/InnerLoopAutopilot/Longitudinal Channel经度通道/PitchStyle/Rate Limiter Dynamic1/Rate Limiter Dynamic with External IC and Autoreset for Change in IC/Unit Delay Resettable External IC/State Control ==

== system simModel2020/PlantModel/B747 Dynamics动力学参数计算/Forces and Moments动力学计算/Compute Body Frame Forces and Moments气动力和力矩/Wind frame F& M 气动力计算/Lateral Channel/Cl/roll factors ==
  p,q,r : Inport
  Airspeed : Inport  Port=2
  Constant : Constant  Value=B747.aero.Clp
      settings: AttributesFormatString=%<Value>
  Constant1 : Constant  Value=B747.aero.Clr
      settings: AttributesFormatString=%<Value>
  Get p : Selector  InputPortWidth=3  IndexOptions=Index vector (dialog)  Indices=1  OutputSizes=[(-2)]
  Get r : Selector  InputPortWidth=3  IndexOptions=Index vector (dialog)  Indices=3  OutputSizes=[(-2)]
  Product : Product  SaturateOnIntegerOverflow=on  OutDataTypeStr=Inherit: Same as first input
  Product1 : Product  SaturateOnIntegerOverflow=on  OutDataTypeStr=Inherit: Same as first input
  roll rate fact : Subsystem
  yaw rate fact : Subsystem
  Clp : Outport
  Clr : Outport  Port=2
  wires:
  Get r/1 -> yaw rate fact/1(r)
  p,q,r/1 -> Get r/1, Get p/1
  Get p/1 -> roll rate fact/1(p)
  Airspeed/1 -> yaw rate fact/2(Airspeed), roll rate fact/2(Airspeed)
  yaw rate fact/1(Yaw Rate Fac) -> Product1/2
  Constant1/1 -> Product1/1
  roll rate fact/1(Roll Rate Fac) -> Product/2
  Constant/1 -> Product/1
  Product1/1 -> Clr/1
  Product/1 -> Clp/1

== system simModel2020/PlantModel/B747 Dynamics动力学参数计算/Forces and Moments动力学计算/Compute Body Frame Forces and Moments气动力和力矩/Wind frame F& M 气动力计算/Lateral Channel/Cn/yaw factors ==
  p,q,r : Inport
  Airspeed : Inport  Port=2
  Constant : Constant  Value=B747.aero.Cnp
      settings: AttributesFormatString=%<Value>
  Constant1 : Constant  Value=B747.aero.Cnr
      settings: AttributesFormatString=%<Value>
  Get p : Selector  InputPortWidth=3  IndexOptions=Index vector (dialog)  Indices=1  OutputSizes=[(-2)]
  Get r : Selector  InputPortWidth=3  IndexOptions=Index vector (dialog)  Indices=3  OutputSizes=[(-2)]
  Product : Product  SaturateOnIntegerOverflow=on  OutDataTypeStr=Inherit: Same as first input
  Product1 : Product  SaturateOnIntegerOverflow=on  OutDataTypeStr=Inherit: Same as first input
  roll rate fact : Subsystem
  yaw rate fact : Subsystem
  Cnp : Outport
  Cnr : Outport  Port=2
  wires:
  Airspeed/1 -> yaw rate fact/2(Airspeed), roll rate fact/2(Airspeed)
  Get r/1 -> yaw rate fact/1(r)
  p,q,r/1 -> Get r/1, Get p/1
  Get p/1 -> roll rate fact/1(p)
  roll rate fact/1(Roll Rate Fac) -> Product/2
  Constant/1 -> Product/1
  yaw rate fact/1(Yaw Rate Fac) -> Product1/2
  Constant1/1 -> Product1/1
  Product1/1 -> Cnr/1
  Product/1 -> Cnp/1
